simulink model "adaptive"  (R2021b)
settings: Solver=VariableStepAuto  StartTime=0.0  StopTime=30  RelTol=1e-3
libraries: simulink x2
settings Model: Creator=84232  LastModifiedBy=84232

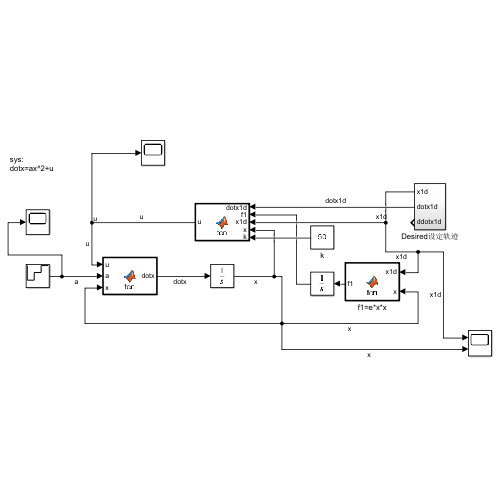
[thumbnail: Simulink's stored preview of the top-level diagram]
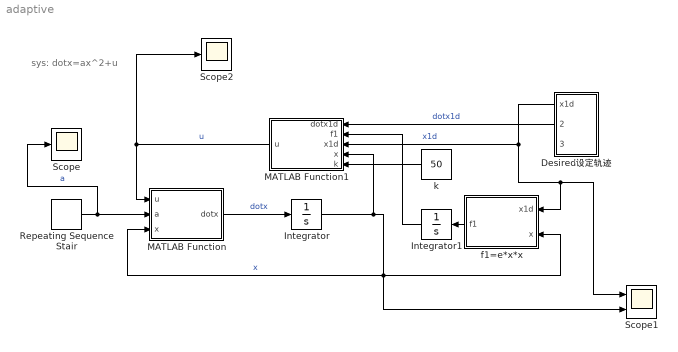
== system adaptive ==
  note: sys:
      | dotx=ax^2+u
  Desired设定轨迹 : Subsystem
  Integrator : Integrator
  Integrator1 : Integrator
  MATLAB Function : MATLAB Function  TreatAsAtomicUnit=on
  MATLAB Function1 : MATLAB Function  TreatAsAtomicUnit=on
  Repeating Sequence Stair : simulink/Sources/Repeating Sequence Stair  OutValues=[1,2,3,].'  tsamp=5  OutMin=[]  OutMax=[]  OutDataTypeStr=double  OutputDataTypeScalingMode=double  OutDataType=fixdt(0,8)  ConRadixGroup=Best Precision: Vector-wise  OutScaling=2^-12
  Scope : Scope
  Scope1 : Scope  NumInputPorts=2
  Scope2 : Scope
  f1=e*x*x : MATLAB Function  TreatAsAtomicUnit=on
  k : Constant  Value=50
  wires:
  MATLAB Function/1(dotx) -> Integrator/1  "dotx"
  Integrator/1 -> MATLAB Function1/4(x), Scope1/2, f1=e*x*x/2(x), MATLAB Function/3(x)  "x"
  Desired设定轨迹/2(dotx1d) -> MATLAB Function1/1(dotx1d)  "dotx1d"
  Repeating Sequence Stair/1 -> Scope/1, MATLAB Function/2(a)  "a"
  MATLAB Function1/1(u) -> MATLAB Function/1(u), Scope2/1  "u"
  k/1 -> MATLAB Function1/5(k)
  Desired设定轨迹/1(x1d) -> MATLAB Function1/3(x1d), Scope1/1, f1=e*x*x/1(x1d)  "x1d"
  f1=e*x*x/1(f1) -> Integrator1/1
  Integrator1/1 -> MATLAB Function1/2(f1)

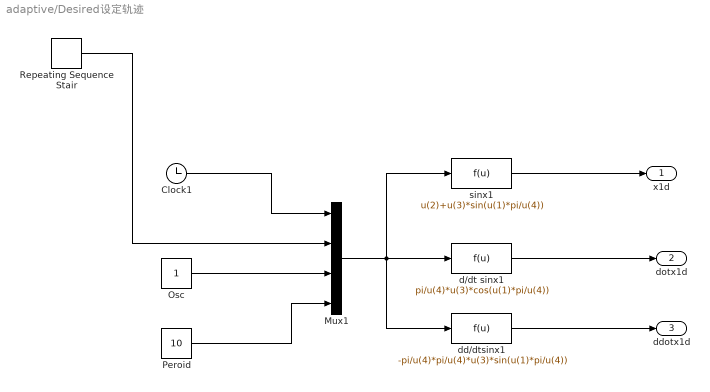
== system adaptive/Desired设定轨迹 ==
  Clock1 : Clock
      settings: Decimation=100
  Mux1 : Mux
  Osc : Constant
  Peroid : Constant  Value=10
  Repeating Sequence Stair : simulink/Sources/Repeating Sequence Stair  OutValues=[1].'  tsamp=10  OutMin=[]  OutMax=[]  OutDataTypeStr=double  OutputDataTypeScalingMode=double  OutDataType=fixdt(0,8)  ConRadixGroup=Best Precision: Vector-wise  OutScaling=2^-12
  d/dt sinx1 : Fcn  Expr=pi/u(4)*u(3)*cos(u(1)*pi/u(4))
  dd/dtsinx1 : Fcn  Expr=-pi/u(4)*pi/u(4)*u(3)*sin(u(1)*pi/u(4))
  sinx1 : Fcn  Expr=u(2)+u(3)*sin(u(1)*pi/u(4))
  x1d : Outport
  dotx1d : Outport  Port=2
  ddotx1d : Outport  Port=3
  wires:
  Repeating Sequence Stair/1 -> Mux1/2
  Clock1/1 -> Mux1/1
  Mux1/1 -> sinx1/1, dd/dtsinx1/1, d/dt sinx1/1
  Osc/1 -> Mux1/3
  Peroid/1 -> Mux1/4
  d/dt sinx1/1 -> dotx1d/1
  dd/dtsinx1/1 -> ddotx1d/1
  sinx1/1 -> x1d/1

== matlab function adaptive/MATLAB Function1 ==
  data: dotx1d input; f1 input; u output; x1d input; x input; k input
function u = fcn(dotx1d,f1,x1d,x,k)
e=x1d-x
u=dotx1d+x*x*f1+k*e

== matlab function adaptive/MATLAB Function ==
  data: u input; dotx output; a input; x input
function dotx = fcn(u,a,x)

dotx=a*x*x+u

== matlab function adaptive/f1=e*x*x ==
  data: x1d input; f1 output; x input
function f1 = fcn(x1d,x)
e=x1d-x
f1=e*x*x
